simulink model "getSpeed"  (R2019a)
settings: Solver=VariableStepAuto  StartTime=0.0  StopTime=10.0  RelTol=1e-3
settings Model: Creator=rahelrickenbach  LastModifiedBy=rahelrickenbach

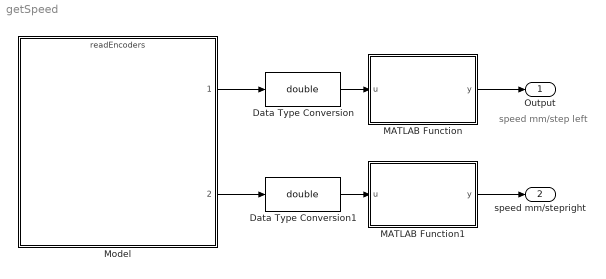
== system getSpeed ==
  note: speed mm/step left
  Data Type Conversion : DataTypeConversion  OutDataTypeStr=double
  Data Type Conversion1 : DataTypeConversion  OutDataTypeStr=double
  MATLAB Function : MATLAB Function  TreatAsAtomicUnit=on
  MATLAB Function1 : MATLAB Function  TreatAsAtomicUnit=on
  Model : ModelReference  ModelNameDialog=readEncoders  SimulationMode=Normal  ModelReferenceVersion=1.6
  Output : Outport
  "speed mm/stepright " : Outport  Port=2
  wires:
  Model/1 -> Data Type Conversion/1
  Model/2 -> Data Type Conversion1/1
  MATLAB Function/1(y) -> Output/1
  MATLAB Function1/1(y) -> "speed mm/stepright "/1
  Data Type Conversion/1 -> MATLAB Function/1(u)
  Data Type Conversion1/1 -> MATLAB Function1/1(u)

== matlab function getSpeed/MATLAB Function1 ==
  data: u input; y output
function y = distanceperstep(u)
% set GearRatio (g) of the following table:
%Gearmotor  30:1	50:1	75:1
%External
%Gearbox
%49:17      0.24	0.14	0.10
%47:19      0.28	0.16	0.11
%45:21      0.33	0.19	0.13
%43:23      0.38	0.22	0.15
%41:25      0.43	0.25	0.17

g = 0.13;
d = 0.8;

distanceperstep = d*pi/(12*g);
u = distanceperstep;

y = u;

== matlab function getSpeed/MATLAB Function ==
  data: u input; y output
function y = distanceperstep(u)
% set GearRatio (g) of the following table:
%Gearmotor  30:1	50:1	75:1
%External
%Gearbox
%49:17      0.24	0.14	0.10
%47:19      0.28	0.16	0.11
%45:21      0.33	0.19	0.13
%43:23      0.38	0.22	0.15
%41:25      0.43	0.25	0.17

g = 0.13;
d = 0.8;

distanceperstep = d*pi/(12*g);
u = distanceperstep;

y = u;
